simulink library "LoadOthers"  (R2014b)
settings: Solver=ode3  StartTime=0.0  StopTime=10.0  RelTol=1e-3
undefined symbols (not defined in the file): powerFactorHighPriorityLoad, powerFactorLowPriorityLoad, powerHighPriority, powerLowPriority, tHighPriorityLoadLPPowerAvailable, tLowPriorityLoadLPPowerAvailable
libraries: goto x5
settings Model: Creator=torstebo  LastModifiedBy=torstebo

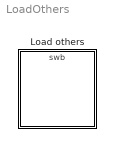
== system LoadOthers ==
  Load others : Subsystem  Tag=Load Others  mask{swbId=1}

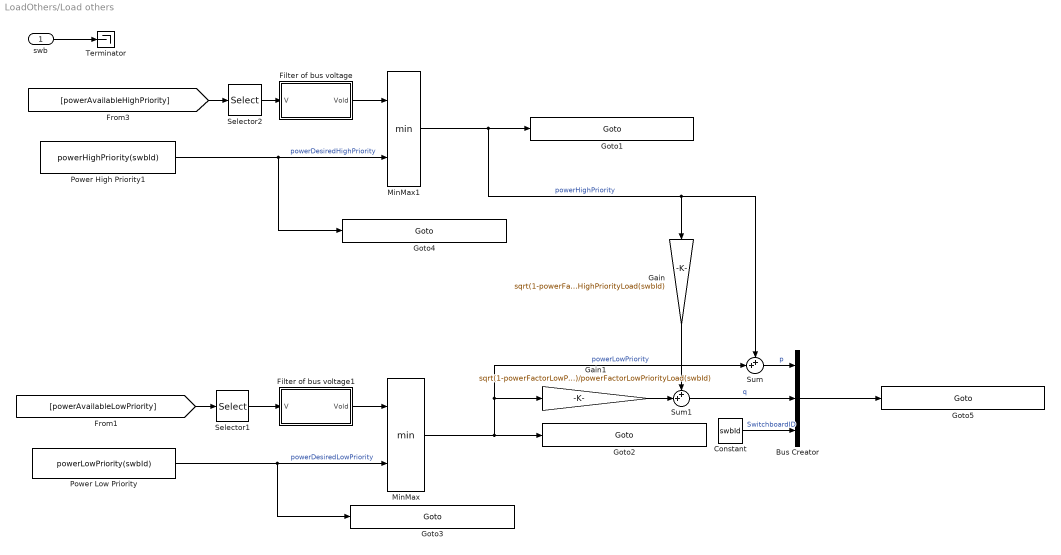
== system LoadOthers/Load others ==
  swb : Inport
  Bus Creator : BusCreator  Inputs='p','q','SwitchboardID'  OutDataTypeStr=Bus: powerLoadsBus  NonVirtualBus=on
  Constant : Constant  Value=swbId
  Filter of bus voltage : Subsystem
  Filter of bus voltage1 : Subsystem
  Gain : Gain  Gain=sqrt(1-powerFactorHighPriorityLoad(swbId)^2)/powerFactorHighPriorityLoad(swbId)
  Gain1 : Gain  Gain=sqrt(1-powerFactorLowPriorityLoad(swbId)^2)/powerFactorLowPriorityLoad(swbId)
  Goto1 : goto/Goto  GotoTag=sprintf('PowerHighPriority%d',swbId)
  Goto2 : goto/Goto  GotoTag=sprintf('PowerLowPriority%d',swbId)
  Goto3 : goto/Goto  GotoTag=sprintf('PowerDesiredLowPriority%d',swbId)
  Goto4 : goto/Goto  GotoTag=sprintf('PowerDesiredHighPriority%d',swbId)
  Goto5 : goto/Goto  GotoTag=sprintf('PowerLoadOthers%d',swbId)
  MinMax : MinMax  Inputs=2  ZeroCross=off
  MinMax1 : MinMax  Inputs=2  ZeroCross=off
  Power High Priority1 : Constant  Value=powerHighPriority(swbId)
  Power Low Priority : Constant  Value=powerLowPriority(swbId)  SampleTime=-1
  Selector1 : Selector  Indices=[swbId]
  Selector2 : Selector  Indices=[swbId]
  Sum : Sum  Inputs=++|
  Sum1 : Sum  Inputs=++|
  Terminator : Terminator
  wires:
  [powerAvailableHighPriority] -> Selector2/1
  [powerAvailableLowPriority] -> Selector1/1
  Constant/1 -> Bus Creator/3  "SwitchboardID"
  Sum1/1 -> Bus Creator/2  "q"
  Sum/1 -> Bus Creator/1  "p"
  Power Low Priority/1 -> Goto3/1, MinMax/2  "powerDesiredLowPriority"
  MinMax/1 -> Goto2/1, Sum/2, Gain1/1  "powerLowPriority"
  Power High Priority1/1 -> Goto4/1, MinMax1/2  "powerDesiredHighPriority"
  Filter of bus voltage/1(Vold) -> MinMax1/1
  Filter of bus voltage1/1(Vold) -> MinMax/1
  Selector2/1 -> Filter of bus voltage/1(V)
  Selector1/1 -> Filter of bus voltage1/1(V)
  Gain/1 -> Sum1/1
  Gain1/1 -> Sum1/2
  MinMax1/1 -> Goto1/1, Gain/1, Sum/1  "powerHighPriority"
  swb/1 -> Terminator/1
  Bus Creator/1 -> Goto5/1

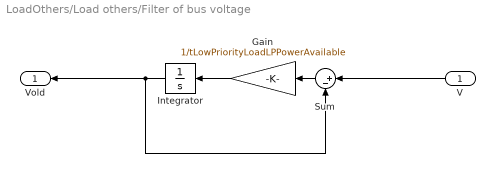
== system LoadOthers/Load others/Filter of bus voltage ==
  V : Inport
  Gain : Gain  Gain=1/tLowPriorityLoadLPPowerAvailable
  Integrator : Integrator  InitialCondition=powerHighPriority(swbId)
  Sum : Sum  Inputs=|+-
  Vold : Outport  PortDimensions=1
  wires:
  Integrator/1 -> Vold/1, Sum/2
  V/1 -> Sum/1
  Sum/1 -> Gain/1
  Gain/1 -> Integrator/1

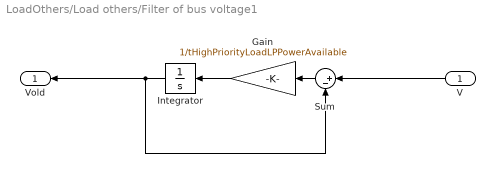
== system LoadOthers/Load others/Filter of bus voltage1 ==
  V : Inport
  Gain : Gain  Gain=1/tHighPriorityLoadLPPowerAvailable
  Integrator : Integrator  InitialCondition=powerLowPriority(swbId)
  Sum : Sum  Inputs=|+-
  Vold : Outport  PortDimensions=1
  wires:
  Integrator/1 -> Vold/1, Sum/2
  V/1 -> Sum/1
  Sum/1 -> Gain/1
  Gain/1 -> Integrator/1
